simulink model "linearization"  (R2017a)
settings: Solver=ode8  StartTime=0.0  StopTime=30  FixedStep=0.01  RelTol=1e-3
settings Model: Creator=manur  LastModifiedBy=manur

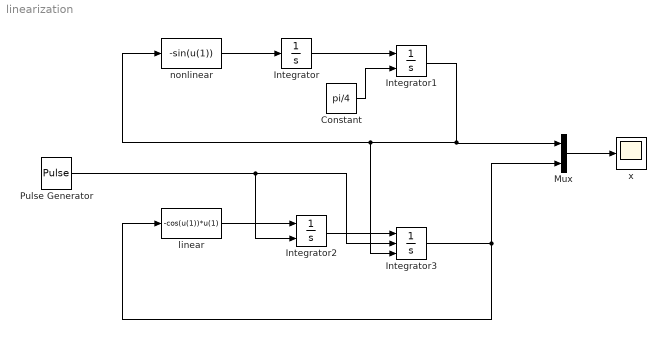
== system linearization ==
  Constant : Constant  Value=pi/4
  Integrator : Integrator
  Integrator1 : Integrator  InitialConditionSource=external  InitialCondition=pi/4
  Integrator2 : Integrator  ExternalReset=rising
  Integrator3 : Integrator  ExternalReset=rising  InitialConditionSource=external  InitialCondition=pi/4
  Mux : Mux  Inputs=2
  Pulse Generator : DiscretePulseGenerator  PulseType=Time based  Period=0.02  PulseWidth=50
  linear : Fcn  Expr=-cos(u(1))*u(1)
  nonlinear : Fcn  Expr=-sin(u(1))
  x : Scope
  wires:
  Integrator/1 -> Integrator1/1
  nonlinear/1 -> Integrator/1
  Integrator1/1 -> Mux/1, Integrator3/3, nonlinear/1
  Integrator3/1 -> Mux/2, linear/1
  Integrator2/1 -> Integrator3/1
  linear/1 -> Integrator2/1
  Mux/1 -> x/1
  Constant/1 -> Integrator1/2
  Pulse Generator/1 -> Integrator2/2, Integrator3/2
